simulink model "trans2"  (R2013a)
settings: Solver=ode45  StartTime=0.0  StopTime=100.0  RelTol=1e-3  AbsTol=1e-6
values from neighbouring files (symbols this model uses):
  A1 = 1    [Kaskady.m]    (also in Kaskady2.m; Palmowski.m = -1/(1-lam1/lam2); transmitacje.m)
  a1 = Aw1*sqrt(2*g*h1max)/h1max    [Kaskady.m]    (also in Kaskady2.m; Skoki.m = 2*Wn*ksi(i); symulek1.m = 1; transmitacje.m)
  A2 = 1    [Kaskady.m]    (also in Kaskady2.m; Palmowski.m = -1-A1; transmitacje.m)
  a2 = Aw2*sqrt(2*g*h2max)/h2max    [Kaskady.m]    (also in Kaskady2.m; Skoki.m = 1; transmitacje.m)
  fwew1 = k(i)*fwew1max    [Kaskady.m]    (also in Kaskady2.m = 0.1; transmitacje.m = 0)
  fwew2 = 0.1    [Kaskady.m]    (also in Kaskady2.m = k(i)*fwew2max; transmitacje.m = 0)
  t0 = 1    [Kaskady.m]    (also in Kaskady2.m; Skoki.m = 0; symulek1.m; transmitacje.m)
settings Model: Creator=LAB320-1552  LastModifiedBy=LAB320-1552
settings DebuggingCC: SolverPrmCheckMsg=none

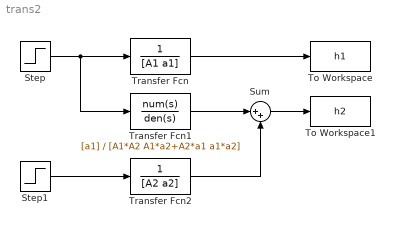
== system trans2 ==
  Step : Step  Time=t0  Before=fwew1  SampleTime=0
  Step1 : Step  Time=t0  Before=fwew2  SampleTime=0
  Sum : Sum  Inputs=|++
  To Workspace : ToWorkspace  VariableName=h1  SampleTime=-1
  To Workspace1 : ToWorkspace  VariableName=h2  SampleTime=-1
  Transfer Fcn : TransferFcn  Denominator=[A1 a1]
  Transfer Fcn1 : TransferFcn  Numerator=[a1]  Denominator=[A1*A2 A1*a2+A2*a1 a1*a2]
  Transfer Fcn2 : TransferFcn  Denominator=[A2 a2]
  wires:
  Step/1 -> Transfer Fcn1/1, Transfer Fcn/1
  Step1/1 -> Transfer Fcn2/1
  Transfer Fcn1/1 -> Sum/1
  Transfer Fcn2/1 -> Sum/2
  Transfer Fcn/1 -> To Workspace/1
  Sum/1 -> To Workspace1/1
